simulink model "MsgEthernetMdl"  (R2022a)
settings: Solver=VariableStepAuto  StartTime=0.0  StopTime=30  FixedStep=1  MaxStep=Inf  RelTol=1e-3  EnableMultiTasking=on
PreLoadFcn:
  | load ethernetTypes.mat;
InitFcn:
  | BitRate = 10e6;
values from neighbouring files (symbols this model uses):
  n = length(stations)    [ethernetHubMask.m]
undefined symbols (not defined in the file or in its folder): gateControl, m, networkselector
libraries: matrix_library x4
(part 2 of 2)

== stateflow chart MsgEthernetMdl/Computer 1/Ethernet Interface 1/CSMA//CD ==
  settings: enableNonTerminalStates=1
  state Standby
    en:
    IsIdle.data = 1;
    send(IsIdle);
    compUtil(1);
  state Receiving
    en:
    delay = RxIn.data.TxDelay;
    err = RxIn.data.CRC;
    forward(RxIn, Rx);
    IsIdle.data = 0;
    send(IsIdle);
    compUtil(0);
  state Transmitting
    en:
    delay = TxIn.data.TxDelay;
    forward(TxIn, TxBuffer);
    IsIdle.data = 0;
    send(IsIdle);
    compUtil(0);
  state Collision
    en:
    n = n + 1;
  state TxSuccess
  state RxSuccess
  state RxFail
  state TxReset
  state RxReset
  (default) -> Standby : {InitRand(); n = 0;}
  TxReset -> Standby
  RxReset -> Standby
  Standby -> Receiving [order 2] : RxIn
  Standby -> Transmitting [order 1] : TxIn
  Transmitting -> TxSuccess [order 1] : after(delay, sec)
  Transmitting -> Collision [order 2] : RxIn[RxIn.data.TxAddress ~= StationID]
  Receiving -> RxFail [order 1] : RxIn
  Receiving -> (junction 14) [order 2] : after(delay, sec)
  (junction 14) -> RxFail [order 2]
  (junction 14) -> RxSuccess [order 1] : [err == 0]
  TxSuccess -> TxReset : TxBuffer
      | {n = 0; TxNext.data=1;
      | send(TxNext);}
  RxSuccess -> (junction 1) : Rx
  RxFail -> RxReset : Rx
  Collision -> (junction 7) : TxBuffer
  (junction 1) -> RxReset [order 1] : [Rx.data.RxAddress == StationID]
      | {DataOut.data = Rx.data.Data;
      | Size = Rx.data.PayloadSize;
      | send(DataOut);}
  (junction 1) -> RxReset [order 2]
  (junction 7) -> TxReset [order 2] : {n = 0;TxNext.data=1;
      |  send(TxNext);}
  (junction 7) -> TxReset [order 1] : [n<16] {TxBuffer.data.BackoffTime = Backoff(n);
      |              forward(TxBuffer, TxRe);}
  data: u function_input; t function_output; IsIdle output double size=1; TxRe output Bus: ethernetPacket size=1; TxNext output double size=1; TxIn input Bus: ethernetPacket size=1; DataOut output Bus: dataPacket size=1; RxIn input Bus: ethernetPacket size=1; delay local double size=1; n local double size=1; TxBuffer local Bus: ethernetPacket size=1; Rx local Bus: ethernetPacket size=1; err local double; StationID parameter; Size output double size=1
  function t = Backoff(u):
    | function t = Backoff(u)
    | t = floor(rand*(2^min([u,10])))*5.12e-5;
  function InitRand:
    | function InitRand
    | rand('seed', StationID);

== matlab function MsgEthernetMdl/Computer 3/Subsystem/Generate Data 1 ==
  data: Data output; PayloadSize output
function [Data, PayloadSize] = randomLengthPayload()
% Generate Ethernet payload of random length between min and max frame size
PayloadSize = 45+randi(1455); % Payload length is 46-1500 bytes
Data = zeros(1,1500);
Data(1:PayloadSize) = randi(3,1, PayloadSize)-1; % Payload values are random (0-255) for a byte

== stateflow chart MsgEthernetMdl/Computer 3/Ethernet Interface 1/CSMA//CD ==
  settings: enableNonTerminalStates=1
  state Standby
    en:
    IsIdle.data = 1;
    send(IsIdle);
    compUtil(1);
  state Receiving
    en:
    delay = RxIn.data.TxDelay;
    err = RxIn.data.CRC;
    forward(RxIn, Rx);
    IsIdle.data = 0;
    send(IsIdle);
    compUtil(0);
  state Transmitting
    en:
    delay = TxIn.data.TxDelay;
    forward(TxIn, TxBuffer);
    IsIdle.data = 0;
    send(IsIdle);
    compUtil(0);
  state Collision
    en:
    n = n + 1;
  state TxSuccess
  state RxSuccess
  state RxFail
  state TxReset
  state RxReset
  (default) -> Standby : {InitRand(); n = 0;}
  TxReset -> Standby
  RxReset -> Standby
  Standby -> Receiving [order 2] : RxIn
  Standby -> Transmitting [order 1] : TxIn
  Transmitting -> TxSuccess [order 1] : after(delay, sec)
  Transmitting -> Collision [order 2] : RxIn[RxIn.data.TxAddress ~= StationID]
  Receiving -> RxFail [order 1] : RxIn
  Receiving -> (junction 14) [order 2] : after(delay, sec)
  (junction 14) -> RxFail [order 2]
  (junction 14) -> RxSuccess [order 1] : [err == 0]
  TxSuccess -> TxReset : TxBuffer
      | {n = 0; TxNext.data=1;
      | send(TxNext);}
  RxSuccess -> (junction 1) : Rx
  RxFail -> RxReset : Rx
  Collision -> (junction 7) : TxBuffer
  (junction 1) -> RxReset [order 1] : [Rx.data.RxAddress == StationID]
      | {DataOut.data = Rx.data.Data;
      | Size = Rx.data.PayloadSize;
      | send(DataOut);}
  (junction 1) -> RxReset [order 2]
  (junction 7) -> TxReset [order 2] : {n = 0;TxNext.data=1;
      |  send(TxNext);}
  (junction 7) -> TxReset [order 1] : [n<16] {TxBuffer.data.BackoffTime = Backoff(n);
      |              forward(TxBuffer, TxRe);}
  data: u function_input; t function_output; IsIdle output double size=1; TxRe output Bus: ethernetPacket size=1; TxNext output double size=1; TxIn input Bus: ethernetPacket size=1; DataOut output Bus: dataPacket size=1; RxIn input Bus: ethernetPacket size=1; delay local double size=1; n local double size=1; TxBuffer local Bus: ethernetPacket size=1; Rx local Bus: ethernetPacket size=1; err local double; StationID parameter; Size output double size=1
  function t = Backoff(u):
    | function t = Backoff(u)
    | t = floor(rand*(2^min([u,10])))*5.12e-5;
  function InitRand:
    | function InitRand
    | rand('seed', StationID);

== matlab function MsgEthernetMdl/Computer 1/Ethernet Interface 1/Simulink Function1/MATLAB Function1 ==
  data: t input; util output; isIdle input
function util = fcn(t, isIdle)

persistent lastTime lastState totalUse;

if isempty(lastTime)
    lastTime = 0;
    lastState = 0;
    totalUse = 0;
end

if lastState ==1 % busy
    totalUse = totalUse + (t - lastTime);
end
lastTime = t;
if isIdle
    lastState = 0;
else
    lastState = 1;
end
if t > 0
    util = totalUse/t;
else
    util = lastState;
end

== matlab function MsgEthernetMdl/Computer 3/Ethernet Interface 1/Simulink Function1/MATLAB Function1 ==
  data: t input; util output; isIdle input
function util = fcn(t, isIdle)

persistent lastTime lastState totalUse;

if isempty(lastTime)
    lastTime = 0;
    lastState = 0;
    totalUse = 0;
end

if lastState ==1 % busy
    totalUse = totalUse + (t - lastTime);
end
lastTime = t;
if isIdle
    lastState = 0;
else
    lastState = 1;
end
if t > 0
    util = totalUse/t;
else
    util = lastState;
end

== stateflow chart MsgEthernetMdl/Computer 4/Ethernet Interface 1/CSMA//CD ==
  settings: enableNonTerminalStates=1
  state Standby
    en:
    IsIdle.data = 1;
    send(IsIdle);
    compUtil(1);
  state Receiving
    en:
    delay = RxIn.data.TxDelay;
    err = RxIn.data.CRC;
    forward(RxIn, Rx);
    IsIdle.data = 0;
    send(IsIdle);
    compUtil(0);
  state Transmitting
    en:
    delay = TxIn.data.TxDelay;
    forward(TxIn, TxBuffer);
    IsIdle.data = 0;
    send(IsIdle);
    compUtil(0);
  state Collision
    en:
    n = n + 1;
  state TxSuccess
  state RxSuccess
  state RxFail
  state TxReset
  state RxReset
  (default) -> Standby : {InitRand(); n = 0;}
  TxReset -> Standby
  RxReset -> Standby
  Standby -> Receiving [order 2] : RxIn
  Standby -> Transmitting [order 1] : TxIn
  Transmitting -> TxSuccess [order 1] : after(delay, sec)
  Transmitting -> Collision [order 2] : RxIn[RxIn.data.TxAddress ~= StationID]
  Receiving -> RxFail [order 1] : RxIn
  Receiving -> (junction 14) [order 2] : after(delay, sec)
  (junction 14) -> RxFail [order 2]
  (junction 14) -> RxSuccess [order 1] : [err == 0]
  TxSuccess -> TxReset : TxBuffer
      | {n = 0; TxNext.data=1;
      | send(TxNext);}
  RxSuccess -> (junction 1) : Rx
  RxFail -> RxReset : Rx
  Collision -> (junction 7) : TxBuffer
  (junction 1) -> RxReset [order 1] : [Rx.data.RxAddress == StationID]
      | {DataOut.data = Rx.data.Data;
      | Size = Rx.data.PayloadSize;
      | send(DataOut);}
  (junction 1) -> RxReset [order 2]
  (junction 7) -> TxReset [order 2] : {n = 0;TxNext.data=1;
      |  send(TxNext);}
  (junction 7) -> TxReset [order 1] : [n<16] {TxBuffer.data.BackoffTime = Backoff(n);
      |              forward(TxBuffer, TxRe);}
  data: u function_input; t function_output; IsIdle output double size=1; TxRe output Bus: ethernetPacket size=1; TxNext output double size=1; TxIn input Bus: ethernetPacket size=1; DataOut output Bus: dataPacket size=1; RxIn input Bus: ethernetPacket size=1; delay local double size=1; n local double size=1; TxBuffer local Bus: ethernetPacket size=1; Rx local Bus: ethernetPacket size=1; err local double; StationID parameter; Size output double size=1
  function t = Backoff(u):
    | function t = Backoff(u)
    | t = floor(rand*(2^min([u,10])))*5.12e-5;
  function InitRand:
    | function InitRand
    | rand('seed', StationID);

== matlab function MsgEthernetMdl/Computer 4/Ethernet Interface 1/Simulink Function1/MATLAB Function1 ==
  data: t input; util output; isIdle input
function util = fcn(t, isIdle)

persistent lastTime lastState totalUse;

if isempty(lastTime)
    lastTime = 0;
    lastState = 0;
    totalUse = 0;
end

if lastState ==1 % busy
    totalUse = totalUse + (t - lastTime);
end
lastTime = t;
if isIdle
    lastState = 0;
else
    lastState = 1;
end
if t > 0
    util = totalUse/t;
else
    util = lastState;
end

== matlab function MsgEthernetMdl/   Ethernet1/Simulink Function/MATLAB Function ==
  data: v1 input; idx output; dest input
function idx = fcn(v1,dest)

if(v1(1)==dest(1)&&v1(2)==dest(2)&&v1(3)==dest(3))
    idx=1;
else
    idx=2;
end

== matlab function MsgEthernetMdl/Router1/Simulink Function/MATLAB Function ==
  data: v1 input; idx output; v2 input; dest input
function idx = fcn(v1,v2,dest)

if(v1(1)==dest(1)&&v1(2)==dest(2)&&v1(3)==dest(3))
    idx=1;
elseif(v2(1)==dest(1)&&v2(2)==dest(2)&&v2(3)==dest(3))
    idx=2;
else
    idx=1;
end

== matlab function MsgEthernetMdl/Computer 2/Subsystem/Generate Data 1 ==
  data: Data output; PayloadSize output
function [Data, PayloadSize] = randomLengthPayload()
% Generate Ethernet payload of random length between min and max frame size
PayloadSize = 45+randi(1455); % Payload length is 46-1500 bytes
Data = zeros(1,1500);
Data(1:PayloadSize) = randi(3,1, PayloadSize)-1; % Payload values are random (0-255) for a byte

== matlab function MsgEthernetMdl/Computer 4/Subsystem/Generate Data 1 ==
  data: Data output; PayloadSize output
function [Data, PayloadSize] = randomLengthPayload()
% Generate Ethernet payload of random length between min and max frame size
PayloadSize = 45+randi(1455); % Payload length is 46-1500 bytes
Data = zeros(1,1500);
Data(1:PayloadSize) = randi(3,1, PayloadSize)-1; % Payload values are random (0-255) for a byte

== matlab function MsgEthernetMdl/   Ethernet2/Simulink Function/MATLAB Function ==
  data: v1 input; idx output; dest input
function idx = fcn(v1,dest)

if(v1(1)==dest(1)&&v1(2)==dest(2)&&v1(3)==dest(3))
    idx=1;
else
    idx=2;
end

== matlab function MsgEthernetMdl/Computer 1/Subsystem/Generate Data 1 ==
  data: Data output; PayloadSize output
function [Data, PayloadSize] = randomLengthPayload()
% Generate Ethernet payload of random length between min and max frame size
PayloadSize = 45+randi(1455); % Payload length is 46-1500 bytes
Data = zeros(1,1500);
Data(1:PayloadSize) = randi(3,1, PayloadSize)-1; % Payload values are random (0-255) for a byte

== stateflow chart MsgEthernetMdl/Computer 2/Ethernet Interface 2/CSMA//CD ==
  settings: enableNonTerminalStates=1
  state Standby
    en:
    IsIdle.data = 1;
    send(IsIdle);
    compUtil(1);
  state Receiving
    en:
    delay = RxIn.data.TxDelay;
    err = RxIn.data.CRC;
    forward(RxIn, Rx);
    IsIdle.data = 0;
    send(IsIdle);
    compUtil(0);
  state Transmitting
    en:
    delay = TxIn.data.TxDelay;
    forward(TxIn, TxBuffer);
    IsIdle.data = 0;
    send(IsIdle);
    compUtil(0);
  state Collision
    en:
    n = n + 1;
  state TxSuccess
  state RxSuccess
  state RxFail
  state TxReset
  state RxReset
  (default) -> Standby : {InitRand(); n = 0;}
  TxReset -> Standby
  RxReset -> Standby
  Standby -> Receiving [order 2] : RxIn
  Standby -> Transmitting [order 1] : TxIn
  Transmitting -> TxSuccess [order 1] : after(delay, sec)
  Transmitting -> Collision [order 2] : RxIn[RxIn.data.TxAddress ~= StationID]
  Receiving -> RxFail [order 1] : RxIn
  Receiving -> (junction 14) [order 2] : after(delay, sec)
  (junction 14) -> RxFail [order 2]
  (junction 14) -> RxSuccess [order 1] : [err == 0]
  TxSuccess -> TxReset : TxBuffer
      | {n = 0; TxNext.data=1;
      | send(TxNext);}
  RxSuccess -> (junction 1) : Rx
  RxFail -> RxReset : Rx
  Collision -> (junction 7) : TxBuffer
  (junction 1) -> RxReset [order 1] : [Rx.data.RxAddress == StationID]
      | {DataOut.data = Rx.data.Data;
      | Size = Rx.data.PayloadSize;
      | send(DataOut);}
  (junction 1) -> RxReset [order 2]
  (junction 7) -> TxReset [order 2] : {n = 0;TxNext.data=1;
      |  send(TxNext);}
  (junction 7) -> TxReset [order 1] : [n<16] {TxBuffer.data.BackoffTime = Backoff(n);
      |              forward(TxBuffer, TxRe);}
  data: u function_input; t function_output; IsIdle output double size=1; TxRe output Bus: ethernetPacket size=1; TxNext output double size=1; TxIn input Bus: ethernetPacket size=1; DataOut output Bus: dataPacket size=1; RxIn input Bus: ethernetPacket size=1; delay local double size=1; n local double size=1; TxBuffer local Bus: ethernetPacket size=1; Rx local Bus: ethernetPacket size=1; err local double; StationID parameter; Size output double size=1
  function t = Backoff(u):
    | function t = Backoff(u)
    | t = floor(rand*(2^min([u,10])))*5.12e-5;
  function InitRand:
    | function InitRand
    | rand('seed', StationID);
